simulink model "PID_controller_long_stage3_plot"  (R2019a)
settings: Solver=VariableStepAuto  StartTime=0.0  StopTime=30  FixedStep=1e-3  RelTol=1e-2
values from neighbouring files (symbols this model uses):
  sys = ss(A,B,C,D,'StateName', {'u'; 'w'; 'q'; 'theta'; 'h'}, 'InputName', {'eta';'epsilon'})    [control_system_v01.m]    (also in control_system_v02.m = ss(A,B,C,D,'StateName', {'u'; 'w'; 'q'; 'theta'},          ')
libraries: simulink x2, aerolibactuator x1
settings Model: Creator=tyson  LastModifiedBy=tyson
settings DebuggingCC: InheritedTsInSrcMsg=none

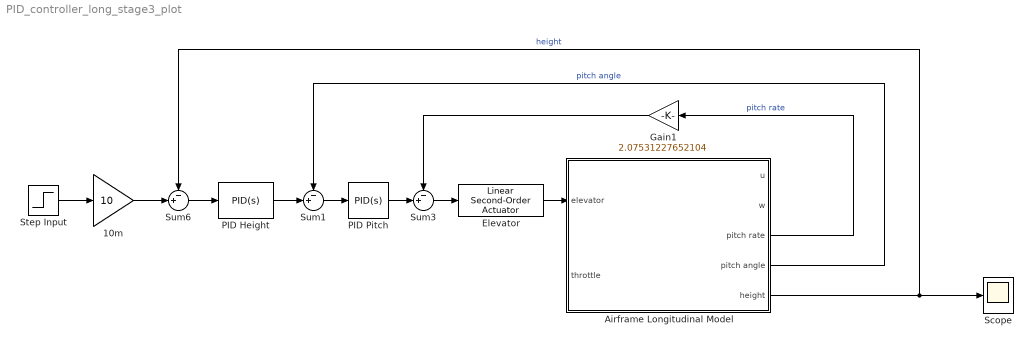
== system PID_controller_long_stage3_plot ==
  10m : Gain  Gain=10
  Airframe Longitudinal Model : Subsystem
      mask Display: image('/home/tyson/Dropbox/Academic/4th Year/ELEN4011/matlab/icons/airframe_long.png');
  Elevator : aerolibactuator/Linear Second-Order Actuator  wn_fin=actuators.naturalFreq  z_fin=actuators.dampingRatio  fin_act_0=0  fin_act_vel=0
      settings: SourceProductName=Aerospace Blockset  SourceProductBaseCode=AE
  Gain1 : Gain  Gain=2.07531227652104
  PID Height : simulink/Continuous/PID Controller  Controller=PID  Form=Parallel  TimeDomain=Continuous-time  SampleTime=-1  IntegratorMethod=Forward Euler  FilterMethod=Forward Euler  ControllerParametersSource=internal  P=0.0203746551941326  I=3.98785899354423e-05  D=-0.014097541537027  UseFilter=on  N=1.21830283710381  TunerSelectOption=Transfer Function Based (PID Tuner App)  InitialConditionSource=internal  InitialConditionForIntegrator=0  InitialConditionForFilter=0  DifferentiatorICPrevScaledInput=0  ExternalReset=none  TrackingMode=off  Kt=1  LimitOutput=on  UpperSaturationLimit=deg2rad(12.5)  LowerSaturationLimit=-deg2rad(12.5)  LinearizeAsGain=on  AntiWindupMode=clamping  Kb=1  POutMin=[]  POutMax=[]  IOutMin=[]  IOutMax=[]  DOutMin=[]  DOutMax=[]  NOutMin=[]  NOutMax=[]  SumOutMin=[]  SumOutMax=[]  SaturationOutMin=[]  SaturationOutMax=[]  PParamMin=[]  PParamMax=[]  IParamMin=[]  IParamMax=[]  DParamMin=[]  DParamMax=[]  NParamMin=[]  NParamMax=[]  KbParamMin=[]  KbParamMax=[]  KtParamMin=[]  KtParamMax=[]  KbOutMin=[]  KbOutMax=[]  KtOutMin=[]  KtOutMax=[]  IntegratorOutMin=[]  IntegratorOutMax=[]  FilterOutMin=[]  FilterOutMax=[]  SumI1OutMin=[]  SumI1OutMax=[]  SumI2OutMin=[]  SumI2OutMax=[]  SumI3OutMin=[]  SumI3OutMax=[]  SumI4OutMin=[]  SumI4OutMax=[]  SumDOutMin=[]  SumDOutMax=[]  DifferentiatorOutMin=[]  DifferentiatorOutMax=[]  FilterDiffOutCoefMin=[]  FilterDiffOutCoefMax=[]  ReciprocalOutMin=[]  ReciprocalOutMax=[]  SumDenOutMin=[]  SumDenOutMax=[]  SumNumOutMin=[]  SumNumOutMax=[]  DivideOutMin=[]  DivideOutMax=[]  IntegratorContinuousStateAttributes=''  IntegratorStateMustResolveToSignalObject=off  IntegratorRTWStateStorageClass=Auto  FilterContinuousStateAttributes=''  FilterStateMustResolveToSignalObject=off  FilterRTWStateStorageClass=Auto  ParallelPVariant=InternalParameters  IdealPVariant=Disabled  IVariant=InternalParameters  DVariant=InternalParameters  IntegratorVariant=Continuous  SatVariant=Enabled  AWVariant=ContClampingParallel  PCopyVariant=Disabled  TRVariant=Disabled  FdbkBlocksVariant=Forward  IdealPFdbkVariant=Disabled  SatFdbkVariant=Disabled  DerivativeFilterVariant=ContFilter  NVariant=InternalParameters  NCopyVariant=Disabled  FilterICVariant=InternalICsFilter  IntegratorICVariant=InternalICs  ExternalResetVariant=Disabled  TRSumVariant=Passthrough  SumFdbkVariant=Disabled  SumVariant=Sum_PID
  PID Pitch : simulink/Continuous/PID Controller  Controller=PID  Form=Parallel  TimeDomain=Continuous-time  SampleTime=-1  IntegratorMethod=Forward Euler  FilterMethod=Forward Euler  ControllerParametersSource=internal  P=11.4841294962751  I=3.73443810245113  D=6.13074519741651  UseFilter=on  N=502.258070962348  TunerSelectOption=Transfer Function Based (PID Tuner App)  InitialConditionSource=internal  InitialConditionForIntegrator=0  InitialConditionForFilter=0  DifferentiatorICPrevScaledInput=0  ExternalReset=none  TrackingMode=off  Kt=1  LimitOutput=off  UpperSaturationLimit=inf  LowerSaturationLimit=-inf  LinearizeAsGain=on  AntiWindupMode=none  Kb=1  POutMin=[]  POutMax=[]  IOutMin=[]  IOutMax=[]  DOutMin=[]  DOutMax=[]  NOutMin=[]  NOutMax=[]  SumOutMin=[]  SumOutMax=[]  SaturationOutMin=[]  SaturationOutMax=[]  PParamMin=[]  PParamMax=[]  IParamMin=[]  IParamMax=[]  DParamMin=[]  DParamMax=[]  NParamMin=[]  NParamMax=[]  KbParamMin=[]  KbParamMax=[]  KtParamMin=[]  KtParamMax=[]  KbOutMin=[]  KbOutMax=[]  KtOutMin=[]  KtOutMax=[]  IntegratorOutMin=[]  IntegratorOutMax=[]  FilterOutMin=[]  FilterOutMax=[]  SumI1OutMin=[]  SumI1OutMax=[]  SumI2OutMin=[]  SumI2OutMax=[]  SumI3OutMin=[]  SumI3OutMax=[]  SumI4OutMin=[]  SumI4OutMax=[]  SumDOutMin=[]  SumDOutMax=[]  DifferentiatorOutMin=[]  DifferentiatorOutMax=[]  FilterDiffOutCoefMin=[]  FilterDiffOutCoefMax=[]  ReciprocalOutMin=[]  ReciprocalOutMax=[]  SumDenOutMin=[]  SumDenOutMax=[]  SumNumOutMin=[]  SumNumOutMax=[]  DivideOutMin=[]  DivideOutMax=[]  IntegratorContinuousStateAttributes=''  IntegratorStateMustResolveToSignalObject=off  IntegratorRTWStateStorageClass=Auto  FilterContinuousStateAttributes=''  FilterStateMustResolveToSignalObject=off  FilterRTWStateStorageClass=Auto  ParallelPVariant=InternalParameters  IdealPVariant=Disabled  IVariant=InternalParameters  DVariant=InternalParameters  IntegratorVariant=Continuous  SatVariant=Disabled  AWVariant=Passthrough  PCopyVariant=Disabled  TRVariant=Disabled  FdbkBlocksVariant=Forward  IdealPFdbkVariant=Disabled  SatFdbkVariant=Disabled  DerivativeFilterVariant=ContFilter  NVariant=InternalParameters  NCopyVariant=Disabled  FilterICVariant=InternalICsFilter  IntegratorICVariant=InternalICs  ExternalResetVariant=Disabled  TRSumVariant=Passthrough  SumFdbkVariant=Disabled  SumVariant=Sum_PID
  Scope : Scope
  Step Input : Step
  Sum1 : Sum  Inputs=-+|
  Sum3 : Sum  Inputs=-+|
  Sum6 : Sum  Inputs=-+|
  wires:
  Elevator/1 -> Airframe Longitudinal Model/1(elevator)
  Airframe Longitudinal Model/3(pitch rate) -> Gain1/1  "pitch rate"
  Sum1/1 -> PID Pitch/1
  PID Pitch/1 -> Sum3/2
  PID Height/1 -> Sum1/2
  Sum6/1 -> PID Height/1
  Sum3/1 -> Elevator/1
  Airframe Longitudinal Model/5(height) -> Sum6/1, Scope/1  "height"
  Step Input/1 -> 10m/1
  Gain1/1 -> Sum3/1
  10m/1 -> Sum6/2
  Airframe Longitudinal Model/4(pitch angle) -> Sum1/1  "pitch angle"

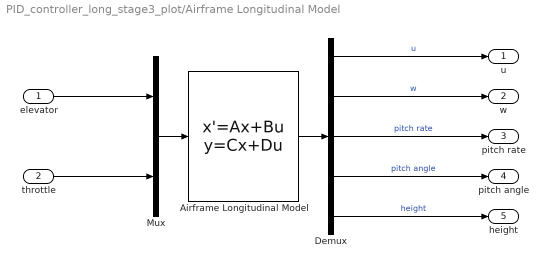
== system PID_controller_long_stage3_plot/Airframe Longitudinal Model ==
  elevator : Inport
  throttle : Inport  Port=2
  Airframe Longitudinal Model : StateSpace  A=sys.long.A  B=sys.long.B  C=sys.long.C  D=sys.long.D  InitialCondition=0
  Demux : Demux  Outputs=5
  Mux : Mux  Inputs=2
  u : Outport
  w : Outport  Port=2
  pitch rate : Outport  Port=3
  pitch angle : Outport  Port=4
  height : Outport  Port=5
  wires:
  throttle/1 -> Mux/2
  Demux/4 -> pitch angle/1  "pitch angle"
  Demux/3 -> pitch rate/1  "pitch rate"
  Mux/1 -> Airframe Longitudinal Model/1
  Airframe Longitudinal Model/1 -> Demux/1
  Demux/1 -> u/1  "u"
  Demux/2 -> w/1  "w"
  Demux/5 -> height/1  "height"
  elevator/1 -> Mux/1
